simulink model "RISaidedCommSys"  (R2024b)
settings: Solver=VariableStepAuto  StartTime=0.0  StopTime=5  RelTol=1e-3
undefined symbols (not defined in the file): doppler, EbNo
libraries: commchan3 x5, commofdm x2, commdigbbndam3 x2, commrandsrc3 x1, commsink2 x1
settings Model: Creator=ravit  LastModifiedBy=ravit
settings DebuggingCC: UnderSpecifiedDimensionMsg=error

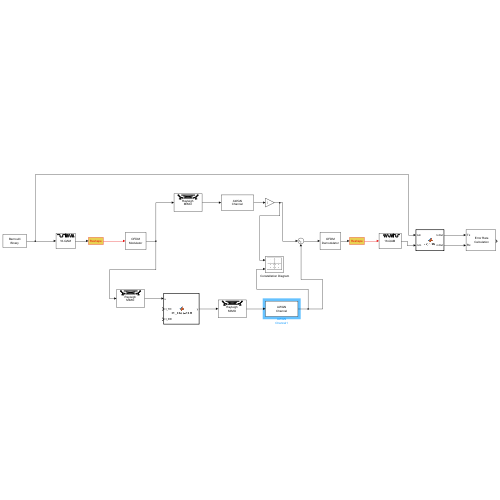
[thumbnail: Simulink's stored preview of the top-level diagram]
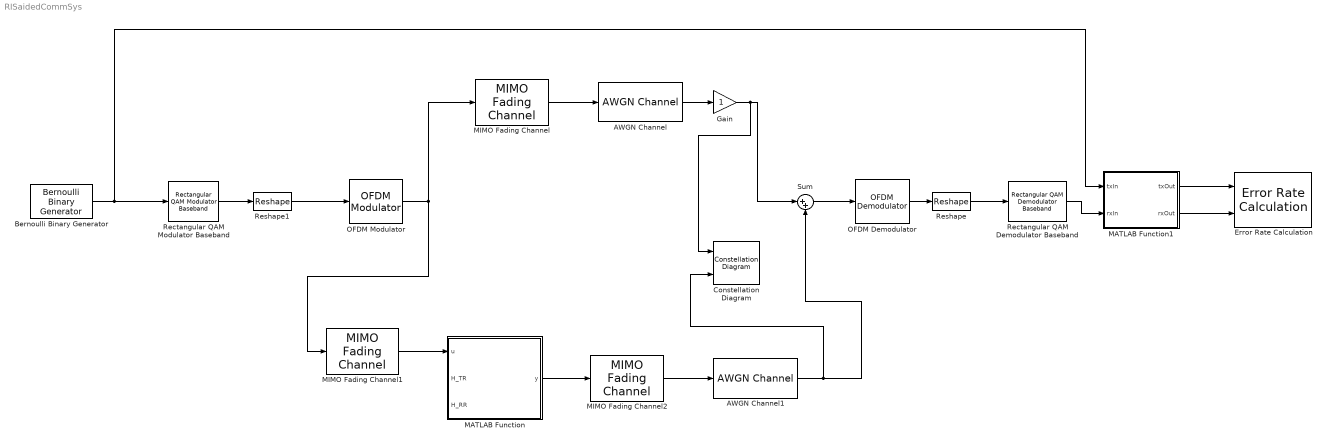
== system RISaidedCommSys ==
  " Constellation Diagram" : ConstellationDiagram  NumInputPorts=2  WindowPosition=[1.000000,1.000000,1536.000000,936.000000,]  ScopeFrameLocation=window  ReferenceConstellation="{[0.7071+0.7071i          -0.7071+0.7071i          -0.7071-0.7071i            0.707-0.7071i][0.7071+0.7071i          -0.7071+0.7071i          -0.7071-0.7071i            0.707-0.7071i]}"  XLimits=[-1.375,1.375]  YLimits=[-1.375,1.375]  ShowLegend=on  MaximizeAxes=off  DefaultConfigurationName=comm.scopes.ConstellationDiagramBlockCfg
  AWGN Channel : commchan3/AWGN Channel  LegacyMode=off  NoiseMethod="Signal to noise ratio  (SNR)"  noiseMode="Signal to noise ratio  (SNR)"  EbNo=10  EsNo=EbNo+10*log10(4)  SNR=15  BitsPerSymbol=1  SignalPower=1  SamplesPerSymbol=1  SymbolPeriod=1  VarianceSource=Parameter  Variance=1  RandomStream=mt19937ar with seed  Seed=4  SimulateUsing=Code generation
  AWGN Channel1 : commchan3/AWGN Channel  LegacyMode=off  NoiseMethod="Signal to noise ratio  (SNR)"  noiseMode="Signal to noise ratio  (SNR)"  EbNo=10  EsNo=10  SNR=15  BitsPerSymbol=1  SignalPower=1  SamplesPerSymbol=1  SymbolPeriod=1  VarianceSource=Parameter  Variance=1  RandomStream=mt19937ar with seed  Seed=4  SimulateUsing=Code generation
  Bernoulli Binary Generator : commrandsrc3/Bernoulli Binary Generator  ProbabilityOfZero=0.5  SeedSource=Auto  Seed=0  SampleTime=1/200  SamplesPerFrame=41600  OutputDataType=single  SimulateUsing=Interpreted execution
  Error Rate Calculation : commsink2/Error Rate Calculation  N=0  st_delay=0  cp_mode=Entire frame  subframe=[]  PMode=Port  WsName=ErrorVec  RsMode2=off  stop=on  numErr=1000  maxBits=1e6
      settings: LibrarySourceBlock=|
      | commhdlsink/Error Rate
      | Calculation
  Gain : Gain
  MATLAB Function : MATLAB Function  TreatAsAtomicUnit=on
  MATLAB Function1 : MATLAB Function  TreatAsAtomicUnit=on
  MIMO Fading Channel : commchan3/MIMO Fading Channel  InheritSampleRate=on  SampleRate=1  PathDelays=1/16000  AveragePathGains=0  NormalizePathGains=on  FadingDistribution=Rayleigh  KFactor=3  DirectPathDopplerShift=0  DirectPathInitialPhase=0  MaximumDopplerShift=2  DopplerSpectrum=doppler('Jakes')  SpatialCorrelationSpecification=None  SpatialCorrelationMatrix=[1 0 0 0; 0 1 0 0; 0 0 1 0; 0 0 0 1]  NumTransmitAntennas=1  NumReceiveAntennas=1  TransmitCorrelationMatrix=[1 0; 0 1]  ReceiveCorrelationMatrix=[1 0; 0 1]  AntennaSelection=Off  NormalizeChannelOutputs=on  PathGainsOutputPort=off  SimulateUsing=Interpreted execution  FadingTechnique=Filtered Gaussian noise  NumSinusoids=48  InitialTimeSource=Property  InitialTime=0  RandomStream=mt19937ar with seed  Seed=73  Visualization=Off  AntennaPairsToDisplay=[ 1, 1 ]  PathsForDopplerDisplay=1  SamplesToDisplay=25%
  MIMO Fading Channel1 : commchan3/MIMO Fading Channel  InheritSampleRate=on  SampleRate=1  PathDelays=0  AveragePathGains=0  NormalizePathGains=on  FadingDistribution=Rayleigh  KFactor=3  DirectPathDopplerShift=0  DirectPathInitialPhase=0  MaximumDopplerShift=5  DopplerSpectrum=doppler('Jakes')  SpatialCorrelationSpecification=None  SpatialCorrelationMatrix=[1 0 0 0; 0 1 0 0; 0 0 1 0; 0 0 0 1]  NumTransmitAntennas=1  NumReceiveAntennas=1  TransmitCorrelationMatrix=[1 0; 0 1]  ReceiveCorrelationMatrix=[1 0; 0 1]  AntennaSelection=Off  NormalizeChannelOutputs=on  PathGainsOutputPort=off  SimulateUsing=Interpreted execution  FadingTechnique=Filtered Gaussian noise  NumSinusoids=48  InitialTimeSource=Property  InitialTime=0  RandomStream=mt19937ar with seed  Seed=73  Visualization=Off  AntennaPairsToDisplay=[ 1, 1 ]  PathsForDopplerDisplay=1  SamplesToDisplay=25%
  MIMO Fading Channel2 : commchan3/MIMO Fading Channel  InheritSampleRate=on  SampleRate=1  PathDelays=0  AveragePathGains=0  NormalizePathGains=on  FadingDistribution=Rayleigh  KFactor=3  DirectPathDopplerShift=0  DirectPathInitialPhase=0  MaximumDopplerShift=2  DopplerSpectrum=doppler('Jakes')  SpatialCorrelationSpecification=None  SpatialCorrelationMatrix=[1 0 0 0; 0 1 0 0; 0 0 1 0; 0 0 0 1]  NumTransmitAntennas=1  NumReceiveAntennas=1  TransmitCorrelationMatrix=[1 0; 0 1]  ReceiveCorrelationMatrix=[1 0; 0 1]  AntennaSelection=Off  NormalizeChannelOutputs=on  PathGainsOutputPort=off  SimulateUsing=Interpreted execution  FadingTechnique=Filtered Gaussian noise  NumSinusoids=48  InitialTimeSource=Property  InitialTime=0  RandomStream=mt19937ar with seed  Seed=73  Visualization=Off  AntennaPairsToDisplay=[ 1, 1 ]  PathsForDopplerDisplay=1  SamplesToDisplay=25%
  OFDM Demodulator : commofdm/OFDM Demodulator  StatePerturbationForJacobian=1.0e-05  FFTLength=64  NumGuardBandCarriers=[6; 5]  RemoveDCCarrier=on  PilotOutputPort=off  PilotCarrierIndices=[12; 26; 40; 54]  CyclicPrefixLength=16  OversamplingFactor=1  NumSymbols=200  NumReceiveAntennas=1  SimulateUsing=Interpreted execution
  OFDM Modulator : commofdm/OFDM Modulator  StatePerturbationForJacobian=1.0e-05  FFTLength=64  NumGuardBandCarriers=[6; 5]  InsertDCNull=on  PilotInputPort=off  PilotCarrierIndices=[12; 26; 40; 54]  CyclicPrefixLength=16  Windowing=off  WindowLength=1  OversamplingFactor=1  NumSymbols=200  NumTransmitAntennas=1  SimulateUsing=Interpreted execution
  Rectangular QAM Demodulator Baseband : commdigbbndam3/Rectangular QAM Demodulator Baseband  M=16  OutType=Bit  DecType=Hard decision  VarSource=Dialog  Variance=1  Dec=Gray  Mapping=[0:15]  PowType=Average Power  MinDist=2  AvgPow=1  PeakPow=1  Ph=0  outDtype1=Inherit via internal rule  outDtype2=Inherit via internal rule  derotateFactorWordLen=16  derotateFactorDataTypeStr=Inherit: Same word length as input  derotateFactorLastDataTypeStr=Inherit: Same word length as input  denormFactorWordLen=16  denormFactorDataTypeStr=Inherit: Same word length as input  denormFactorLastDataTypeStr=Inherit: Same word length as input  prodOutWordLen=32  prodOutOverflowMode=Wrap  prodOutRoundingMode=Floor  prodOutOvFlMode=off  prodOutOvFlModeLastStrValue=off  sumWordLen=32
      settings: LibrarySourceBlock=|
      | commhdldigbbndam/Rectangular QAM
      | Demodulator
      | Baseband
  Rectangular QAM Modulator Baseband : commdigbbndam3/Rectangular QAM Modulator Baseband  M=16  InType=Bit  Enc=Gray  Mapping=[0:15]  PowType=Average Power  MinDist=2  AvgPow=1  PeakPow=1  Ph=0  outDtype=single  outWordLen=16  outUDDataType=sfix(16)  outFracLenMode=Best precision  outFracLen=15  outDataTypeStr=single  outLastDataTypeStr=single
      settings: LibrarySourceBlock=|
      | commhdldigbbndam/Rectangular QAM
      | Modulator
      | Baseband
  Reshape : Reshape  OutputDimensionality=Customize  OutputDimensions=[10400, 1]
  Reshape1 : Reshape  OutputDimensionality=Customize  OutputDimensions=[52, 200]
  Sum : Sum  Inputs=|++
  wires:
  OFDM Modulator/1 -> MIMO Fading Channel1/1, MIMO Fading Channel/1
  MIMO Fading Channel/1 -> AWGN Channel/1
  MIMO Fading Channel2/1 -> AWGN Channel1/1
  MIMO Fading Channel1/1 -> MATLAB Function/1(u)
  MATLAB Function/1(y) -> MIMO Fading Channel2/1
  MATLAB Function1/1(txOut) -> Error Rate Calculation/1
  MATLAB Function1/2(rxOut) -> Error Rate Calculation/2
  Rectangular QAM Demodulator Baseband/1 -> MATLAB Function1/2(rxIn)
  Bernoulli Binary Generator/1 -> Rectangular QAM Modulator Baseband/1, MATLAB Function1/1(txIn)
  AWGN Channel1/1 -> " Constellation Diagram"/2, Sum/2
  AWGN Channel/1 -> Gain/1
  Sum/1 -> OFDM Demodulator/1
  Reshape/1 -> Rectangular QAM Demodulator Baseband/1
  OFDM Demodulator/1 -> Reshape/1
  Reshape1/1 -> OFDM Modulator/1
  Rectangular QAM Modulator Baseband/1 -> Reshape1/1
  Gain/1 -> " Constellation Diagram"/1, Sum/1

== matlab function RISaidedCommSys/MATLAB Function1 ==
  data: txIn input; txOut output; rxIn input; rxOut output
function [txOut, rxOut] = alignBits(txIn, rxIn)
% Align two bit vectors by trimming to the same length.
% txIn, rxIn: column vectors (frame-based)
% txOut, rxOut: trimmed column vectors of equal length

% Ensure column orientation
txIn = txIn(:);
rxIn = rxIn(:);

nTx = numel(txIn);
nRx = numel(rxIn);
n = min(nTx, nRx);

% If no data yet, return empty columns
if n == 0
    txOut = zeros(0,1,'like',txIn);
    rxOut = zeros(0,1,'like',rxIn);
    return;
end

txOut = txIn(1:n);
rxOut = rxIn(1:n);
end

== matlab function RISaidedCommSys/MATLAB Function ==
  data: u input size=16000; y output; H_TR input; H_RR input
function y = RIS_PhaseShift(u, H_TR, H_RR)
% RIS_PhaseShift - Applies optimal phase shifts for RIS-aided communication
% Inputs:
%   u: input signal from OFDM Modulator (can be scalar or vector)
%   H_TR: channel matrix from Transmitter to RIS ([1 x N] vector for N RIS elements)
%   H_RR: channel matrix from RIS to Receiver ([N x 1] vector for N RIS elements)
% Output:
%   y: output signal after applying RIS phase shifts

if size(H_TR, 1) ~= 1
    error('H_TR should be a [1 x N] vector representing channels from transmitter to N RIS elements');
end
if size(H_RR, 2) ~= 1
    error('H_RR should be a [N x 1] vector representing channels from N RIS elements to receiver');
end
if size(H_TR, 2) ~= size(H_RR, 1)
    error('Number of RIS elements must match: H_TR columns must equal H_RR rows');
end

% Get the number of RIS elements
N = size(H_TR, 2);  % or equivalently size(H_RR, 1)

% Calculate optimal phase shifts for coherent combining
% For each RIS element n, the cascaded channel coefficient is H_TR(n) * exp(j*theta_n) * H_RR(n)
% To maximize the received signal power, we want all paths to add constructively
% This means aligning all phase components to the same reference phase

theta_opt = -(angle(H_TR) + angle(H_RR.'));  % Note: H_RR.' to make it [1 x N]

% Ensure theta_opt is a column vector for consistency
theta_opt = theta_opt(:);  % Convert to column vector [N x 1]

RIS_Matrix = diag(exp(1j * theta_opt));

% Mathematical model: y = H_RR^T * RIS_Matrix * H_TR^T * u
y = (H_RR.' * RIS_Matrix * H_TR.') * u;

end

% Example usage and verification function
function example_usage()
    N = 8;  % Number of RIS elements
    
    % Random channel coefficients (complex)
    H_TR = (randn(1, N) + 1j*randn(1, N)) / sqrt(2);
    H_RR = (randn(N, 1) + 1j*randn(N, 1)) / sqrt(2);  
    
    % Input signal
    u = 1;  % Unit amplitude signal for testing
    
    % Apply RIS phase shift
    y_optimized = RIS_PhaseShift(u, H_TR, H_RR);
    
    theta_random = 2*pi*rand(N, 1) - pi;  % Random phases [-pi, pi]
    RIS_random = diag(exp(1j * theta_random));
    y_random = (H_RR.' * RIS_random * H_TR.') * u;
    
    fprintf('Optimized RIS output power: %.4f\n', abs(y_optimized)^2);
    fprintf('Random phase output power: %.4f\n', abs(y_random)^2);
    fprintf('Power gain ratio: %.2f\n', abs(y_optimized)^2 / abs(y_random)^2);
    
    % Verify phase alignment
    theta_opt = -(angle(H_TR) + angle(H_RR.'));
    effective_phases = angle(H_TR) + theta_opt + angle(H_RR.');
    fprintf('Phase alignment check - std of effective phases: %.6f rad\n', std(effective_phases));
end
